simulink model "px4_SDCard_logging"  (R2019b)
settings: Solver=FixedStepAuto  StartTime=0.0  StopTime=20  RelTol=1e-3  EnableMultiTasking=on
libraries: px4uORBlib x1
settings Model: ExtModeTrigDuration=10  Creator=The MathWorks, Inc.  LastModifiedBy=The MathWorks, Inc.
settings SolverCC: PositivePriorityOrder=on
settings OptimizationCC: EnhancedBackFolding=on  PassReuseOutputArgsAs=Individual arguments  ZeroExternalMemoryAtStartup=off  ZeroInternalMemoryAtStartup=off  MaxStackSize=64  OptimizeBlockOrder=speed  DifferentSizesBufferReuse=on  OptimizationCustomize=off  EfficientTunableParamExpr=on
settings DebuggingCC: ParameterTunabilityLossMsg=error
settings HardwareCC: ProdBitPerPointer=32  ProdBitPerSizeT=32  ProdBitPerPtrDiffT=32  ProdLargestAtomicInteger=Long  ProdLargestAtomicFloat=Double  ProdWordSize=32  ProdLongLongMode=on  ProdHWDeviceType=ARM Compatible->ARM Cortex
settings SFSimCC: MATLABDynamicMemAlloc=off
settings RTWCC: SystemTargetFile=ert.tlc  HardwareBoard=PX4 Pixhawk 1  TLCOptions="-aInlineSetEventsForThisBaseRateFcn=TLC_FALSE -aSuppressMultiTaskScheduler=TLC_FALSE  -aRateBasedStepFcn=0"  TemplateMakefile=ert_default_tmf  GenerateReport=on  Toolchain=GNU Tools for PX4 Autopilots  IncludeHyperlinkInReport=on  LaunchReport=on  TargetLang=C++  GenerateTraceInfo=on  GenerateTraceReport=on  GenerateTraceReportSl=on  GenerateTraceReportSf=on  GenerateTraceReportEml=on
settings CodeAppCC: ForceParamTrailComments=on  IgnoreCustomStorageClasses=off  OperatorAnnotations=on  SimulinkDataObjDesc=on  SFDataObjDesc=on  InsertBlockDesc=on

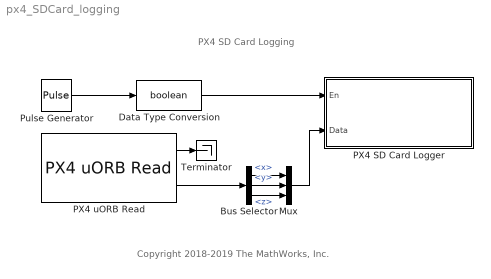
== system px4_SDCard_logging ==
  note: PX4 SD Card Logging
  note: Copyright 2018-2019 The MathWorks, Inc.
  Bus Selector : BusSelector  OutputSignals=x,y,z
  Data Type Conversion : DataTypeConversion  OutDataTypeStr=boolean
  Mux : Mux  Inputs=3
  PX4 SD Card Logger : Subsystem  mask(PX4 SD Card Logger){logfile=/fs/microsd/log, logfilename=accel_data, cacheflag=off, numRecs=100}
      mask prompts: logfile "Log Folder"; logfilename "Log File Name"; cacheflag "Cache in Memory"; numRecs "Maximum Record Count"
      mask help:
      | Log data to a specified file on the SD card
      |
      | The block accepts two inputs, enable and data. The incoming data is logged into the SD card when the enable signal is high and the number of data points logged is less than the Maximum Record Count specified.
      |
      | The specified folder should be present in the SD card for logging.
      |
      | If Cache in Memory is unchecked, the data is written to the SD card at every timestep.  If Cache in Memory is checked, data is cached in the memory and is written to SD card only when enable goes low or when the number of data points logged reaches the Maximum Record Count specified.
      mask init:
      | logname=uint8([logfile,'/',logfilename]);
      mask Help: eval('codertarget.internal.helpView(''px4'',''px4sdcardexample'')');
      mask Display:
      | fprintf([get_param(gcb,'logfile'),'/',get_param(gcb,'logfilename')])
      | port_label('input',1,'en')
      | port_label('input',2,'data')
  PX4 uORB Read : px4uORBlib/PX4 uORB Read  uORBTopic=sensor_accel  sampleTime=-1  BlockingMode=off  BlockTimeout=1e-3
      settings: SourceProductName=Embedded Coder Support Package for PX4 Autopilots  SourceProductBaseCode=PX4AUTOPILOTS
  Pulse Generator : DiscretePulseGenerator  Period=50  PulseWidth=20  SampleTime=0.01  VectorParams1D=off
  Terminator : Terminator
  wires:
  Pulse Generator/1 -> Data Type Conversion/1
  Data Type Conversion/1 -> PX4 SD Card Logger/1(En)
  PX4 uORB Read/1 -> Terminator/1
  Bus Selector/1 -> Mux/1  "<x>"
  Bus Selector/2 -> Mux/2  "<y>"
  PX4 uORB Read/2 -> Bus Selector/1
  Bus Selector/3 -> Mux/3  "<z>"
  Mux/1 -> PX4 SD Card Logger/2(Data)

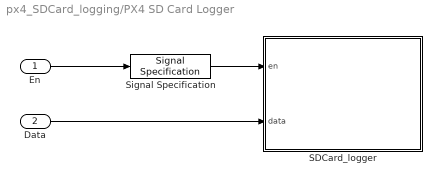
== system px4_SDCard_logging/PX4 SD Card Logger ==
  En : Inport
  Data : Inport  Port=2
  SDCard_logger : MATLAB Function  TreatAsAtomicUnit=on
  Signal Specification : SignalSpecification  OutDataTypeStr=boolean
  wires:
  Signal Specification/1 -> SDCard_logger/1(en)
  En/1 -> Signal Specification/1
  Data/1 -> SDCard_logger/2(data)

== matlab function px4_SDCard_logging/PX4 SD Card Logger/SDCard_logger ==
  data: en input boolean; data input; logname parameter uint8; cacheflag parameter boolean; numRecs parameter uint32
%% PX4 SD Card Logger
% Note: All data needs to be of the same type (e.g. double)
% Header information format:
%           String "MWLOG"
%           Time/Date 4 bytes (time())
%           Number of Signals per record Logged 1 byte (256 max)
%           Data Type of Signals Logged  1 byte (1-10)
%           Number of bytes per record 2 bytes (65535 max)
% This does NOT include the number of data sets logged.
% i.e. The Reader is responsible for reading until EOF.
% Steve Kuznicki
% Copyright 2018 The MathWorks, Inc.

function SDCard_logger(en, data, logname, cacheflag, numRecs)

persistent fp isflushed isopen count  elem_size vect_size datastore timestore count_prev

if coder.target('Rtw')
    
    coder.cinclude('<stdio.h>');
    coder.cinclude('<time.h>');
    
    if coder.target('Rtw')
        coder.cinclude('<drivers/drv_hrt.h>');
    end
    
    if coder.target('Rtw')
        timestamp=coder.opaque('uint64_t');
        timestamp=coder.ceval('hrt_absolute_time');
    else
        timestamp = uint64(0);
    end
    
    if isempty(count)
        count = uint32(0);
        count_prev=count;
        fp = coder.opaque('FILE*', 'NULL');
        isflushed = false;
        if cacheflag == true
            datastore = zeros(numRecs*uint32(coder.const(numel(data))), 1, 'like', data);
            timestore=uint64(zeros(numRecs, 1));
        end
        
        [elsize, eltype] = get_elem_size(data);
        elem_size = coder.const(uint16(elsize));
        elem_type = coder.const(uint8(eltype));
        vect_size = coder.const(uint8(numel(data)));
        coder.ceval('printf',['OPENING file %s vect_size %d elem_size %d numRecs %d %c' uint8(0)], ...
            [logname,'.bin', int8(0)], uint32(vect_size), uint32(elem_size), uint32(numRecs), uint8(10));
        fp = coder.ceval('fopen', [logname,'.bin', int8(0)], ['wb', int8(0)]);
        isopen = true;
        
        % Write header information here
        % header token + version
        mlStrVer = 'MWLOG';
        coder.ceval('fwrite', coder.rref(mlStrVer), uint32(1), length(mlStrVer), fp);
        % date/time
        tm = uint32(0);
        tmptr = uint32(0);
        tm = coder.ceval('time',coder.wref(tmptr));
        coder.ceval('fwrite', coder.rref(tm), uint32(4), uint32(1), fp);
        % number of elements in each record
        coder.ceval('fwrite', coder.rref(vect_size), uint32(1), uint32(1), fp);
        % data type of the elements
        coder.ceval('fwrite', coder.rref(elem_type), uint32(1), uint32(1), fp);
        % size of each record in bytes
        recSize = elem_size * uint16(vect_size);
        coder.ceval('fwrite', coder.rref(recSize), uint32(2), uint32(1), fp);
    end
    
    
    if (en && (count < numRecs))
        
        if isopen == false
            % open file in append mode
            fp = coder.ceval('fopen', [logname,'.bin', int8(0)], ['ab', int8(0)]);
            isflushed = false;
            isopen = true;
            count_prev=count;
        end
        
        % cache data in memory or use fwrite
        if cacheflag == true
            addr = (count*uint32(vect_size))+1;
            for idx = 1:vect_size
                datastore(addr) = data(idx);
                addr = addr + 1;
            end
            timestore(count+uint32(1))=uint64(timestamp);
        else
            coder.ceval('fwrite', coder.rref(data), elem_size, vect_size, fp);
            if coder.target('Rtw')
                coder.ceval('fwrite', coder.rref(timestamp), uint32(8), uint32(1), fp);
            end
        end
        count = count + uint32(1);
        
    else
        if isopen == true
            if ~isflushed
                coder.ceval('printf',['CLOSING file. count = %d %c' uint8(0)], uint32(count), uint8(10));
                if cacheflag
                    for idx=count_prev+1:count
                        for idx2=(idx-1)*double(vect_size)+1:(idx-1)*double(vect_size)+double(vect_size)
                            coder.ceval('fwrite', coder.rref(datastore(idx2)), elem_size, uint32(1), fp);
                        end
                        coder.ceval('fwrite', coder.rref(timestore(idx)), uint32(8), uint32(1), fp);
                    end
                end
                coder.ceval('fflush', fp);
                isflushed = true;
            end
            coder.ceval('fclose', fp);
        end
        isopen = false;
    end
end

% return the size of the element in bytes
    function [elem_size, dtype] = get_elem_size(data)
        switch(class(data))
            case 'double'
                elem_size = 8;
                dtype = 1;
            case 'single'
                elem_size = 4;
                dtype = 2;
            case 'int32'
                elem_size = 4;
                dtype = 3;
            case 'uint32'
                elem_size = 4;
                dtype = 4;
            case 'int16'
                elem_size = 2;
                dtype = 5;
            case 'uint16'
                elem_size = 2;
                dtype = 6;
            case 'int8'
                elem_size = 1;
                dtype = 7;
            case 'uint8'
                elem_size = 1;
                dtype = 8;
            case 'logical'
                elem_size = 1;
                dtype = 9;
            case 'embedded.fi'
                nt = numerictype(data);
                elem_size = 2^ceil(log2(ceil(nt.WordLength / 8)));
                dtype = 10;
        end
        if ~isreal(data)
            elem_size = elem_size*2;
        end
        
        elem_size = uint16(elem_size);
        dtype = uint8(dtype);
    end
end
